simulink model "EHRTC_Block_Diagram"  (R2018b)
settings: Solver=VariableStepAuto  StartTime=0.0  StopTime=12000  RelTol=1e-3
values from neighbouring files (symbols this model uses):
  kc = 125    [EHRTC_initData.m]
  kE = 1000    [EHRTC_initData.m]
  kp = 500    [EHRTC_initData.m]
  Tc = 300    [EHRTC_initData.m]
  Tp = 60    [EHRTC_initData.m]
settings Model: Creator=bogda  LastModifiedBy=bogda

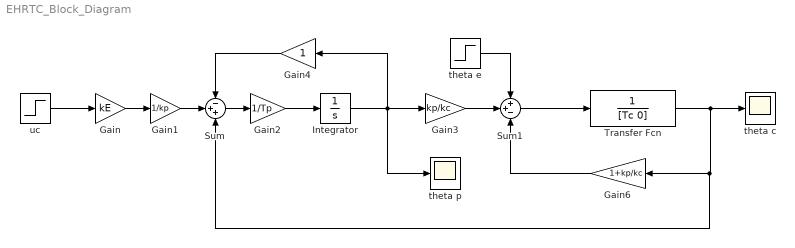
== system EHRTC_Block_Diagram ==
  Gain : Gain  Gain=kE
  Gain1 : Gain  Gain=1/kp
  Gain2 : Gain  Gain=1/Tp
  Gain3 : Gain  Gain=kp/kc
  Gain4 : Gain
  Gain6 : Gain  Gain=1+kp/kc
  Integrator : Integrator
  Sum : Sum  Inputs=-++
  Sum1 : Sum  Inputs=++-
  Transfer Fcn : TransferFcn  Denominator=[Tc 0]
  "theta c " : Scope
  theta e : Step  Time=5000  After=-10  SampleTime=0
  theta p : Scope
  uc : Step  Time=0  After=2.5  SampleTime=0
  wires:
  Gain/1 -> Gain1/1
  Gain1/1 -> Sum/2
  Sum/1 -> Gain2/1
  Integrator/1 -> theta p/1, Gain4/1, Gain3/1
  Gain2/1 -> Integrator/1
  Gain4/1 -> Sum/1
  Gain3/1 -> Sum1/2
  Sum1/1 -> Transfer Fcn/1
  uc/1 -> Gain/1
  theta e/1 -> Sum1/1
  Gain6/1 -> Sum1/3
  Transfer Fcn/1 -> Sum/3, Gain6/1, "theta c "/1
